simulink model "Drone"  (R2014a)
settings: Solver=ode45  StartTime=0.0  StopTime=10.0  RelTol=1e-3
libraries: mpclib x1
settings Model: Creator=jerry  LastModifiedBy=student
settings DebuggingCC: UnderspecifiedInitializationDetection=Classic

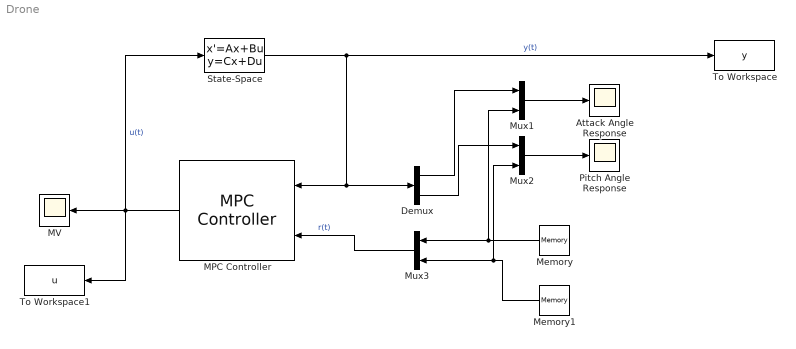
== system Drone ==
  Attack Angle Response : Scope
      settings: SaveName=ScopeData5
  Demux : Demux  Outputs=2
  MPC Controller : mpclib/MPC Controller  mpcobj=MPC Controller  x0=[]  md_inport=off  mv_inport=off  lims_inport=off  switch_inport=off  ywt_inport=off  duwt_inport=off  rhoeps_inport=off  cost_outport=off  return_sequence=off  return_qpstatus=off  is_multiple=0  enable_value=0  n_mv=1  n_mo=2  n_md=0  n_ts=1  is_designfromscratch=0  BlockDataType=double  SampleTimeInherited=off  ref_from_ws=off  ref_signal_name=[]  ref_preview=off  md_from_ws=off  md_signal_name=[]  md_preview=off  from_project=off  project_file=MPCtask.mat
  MV : Scope
      settings: SaveName=ScopeData4
  Memory : Memory
  Memory1 : Memory
  Mux1 : Mux  Inputs=2
  Mux2 : Mux  Inputs=2
  Mux3 : Mux  Inputs=2
  Pitch Angle Response : Scope
      settings: SaveName=ScopeData7
  State-Space : StateSpace  X0=0
  To Workspace : ToWorkspace  VariableName=y  SaveFormat=Timeseries  SampleTime=-1
  To Workspace1 : ToWorkspace  VariableName=u  SaveFormat=Timeseries  SampleTime=-1
  wires:
  State-Space/1 -> To Workspace/1, MPC Controller/1, Demux/1  "y(t)"
  MPC Controller/1 -> To Workspace1/1, State-Space/1, MV/1  "u(t)"
  Mux1/1 -> Attack Angle Response/1
  Mux2/1 -> Pitch Angle Response/1
  Demux/1 -> Mux1/1
  Demux/2 -> Mux2/1
  Mux3/1 -> MPC Controller/2  "r(t)"
  Memory/1 -> Mux1/2, Mux3/1
  Memory1/1 -> Mux2/2, Mux3/2
